simulink library "ERRORS"  (R2021b)
settings: Solver=VariableStepAuto  StartTime=0.0  StopTime=10.0  RelTol=1e-3
settings Model: Creator=Davide  LastModifiedBy=Davide

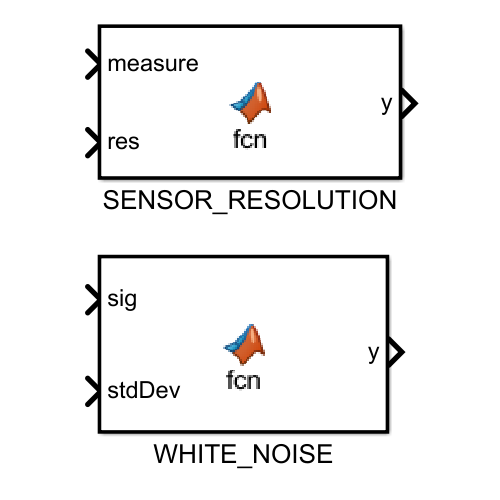
[thumbnail: Simulink's stored preview of the top-level diagram]
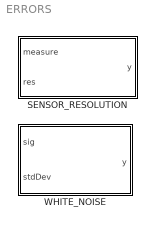
== system ERRORS ==
  SENSOR_RESOLUTION : MATLAB Function  TreatAsAtomicUnit=on
  WHITE_NOISE : MATLAB Function  TreatAsAtomicUnit=on

== matlab function ERRORS/WHITE_NOISE ==
  data: sig input; y output; stdDev input
function y = fcn(sig,stdDev)

y = sig + randn(size(stdDev)).*stdDev;

== matlab function ERRORS/SENSOR_RESOLUTION ==
  data: measure input; y output; res input
function y = fcn(measure,res)

y = round(measure/res)*res;
